simulink model "carstateflow"  (R2020b)
settings: Solver=FixedStepAuto  StartTime=0.0  StopTime=2.2  FixedStep=0.1  RelTol=1e-3
settings Model: Creator=yuto  LastModifiedBy=yuto

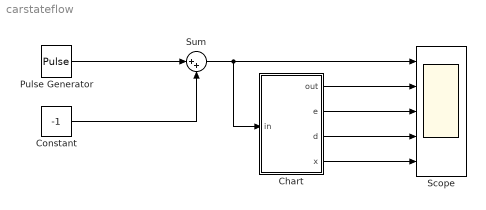
== system carstateflow ==
  Chart : Stateflow chart  TreatAsAtomicUnit=on
  Constant : Constant  Value=-1
  Pulse Generator : DiscretePulseGenerator  PulseType=Time based  Amplitude=2  PulseWidth=50
  Scope : Scope  NumInputPorts=5
  Sum : Sum  Inputs=|++
  wires:
  Pulse Generator/1 -> Sum/1
  Constant/1 -> Sum/2
  Sum/1 -> Chart/1(in), Scope/1
  Chart/1(out) -> Scope/2
  Chart/2(e) -> Scope/3
  Chart/3(d) -> Scope/4
  Chart/4(x) -> Scope/5

== stateflow chart carstateflow/Chart ==
  state st2
    entry:
    out = 2;
    e = 1;
    during:
    d = d + 1;
    exit:
    x = 1;
  state st3
    entry:
    out = 3;
    e = -1;
    during:
    d = d - 1;
    exit:
    x = -1;
  state st1
    entry:
    out = 1
    e = 0;
    d = 0;
    x = 0;
  (default) -> st1
  st2 -> st3
  st1 -> st2
  data: in input; out output; e output; d output; x output
